simulink model "traffic_light_with_urgent_manger"  (R2020a)
settings: Solver=FixedStepDiscrete  StartTime=0.0  StopTime=12  FixedStep=1e-3  RelTol=1e-3
settings Model: Creator=Administrator  LastModifiedBy=Administrator
settings OptimizationCC: DefaultParameterBehavior=Inlined  UseDivisionForNetSlopeComputation=on  GainParamInheritBuiltInType=on  UseFloatMulNetSlope=on  InlineInvariantSignals=on  PassReuseOutputArgsAs=Individual arguments  ZeroExternalMemoryAtStartup=off  ZeroInternalMemoryAtStartup=off  NoFixptDivByZeroProtection=on  EfficientFloat2IntCast=on  LifeSpan=1  OptimizeBlockOrder=speed  DifferentSizesBufferReuse=on  EfficientTunableParamExpr=on
settings DebuggingCC: ParameterTunabilityLossMsg=error
settings HardwareCC: ProdBitPerInt=16  ProdBitPerPointer=16  ProdBitPerSizeT=16  ProdBitPerPtrDiffT=16  ProdLargestAtomicFloat=None  ProdWordSize=8  ProdLongLongMode=on  ProdHWDeviceType=Atmel->AVR
settings SFSimCC: MATLABDynamicMemAlloc=off
settings RTWCC: SystemTargetFile=ert.tlc  TemplateMakefile=ert_default_tmf  PortableWordSizes=on
settings CodeAppCC: ForceParamTrailComments=on  IgnoreCustomStorageClasses=off  OperatorAnnotations=on  SimulinkDataObjDesc=on  SFDataObjDesc=on  CustomSymbolStrGlobalVar=rt$N$M  CustomSymbolStrType=$N$M  CustomSymbolStrFcn=$N$M$F  CustomSymbolStrMacro=$N$M  InsertBlockDesc=on
settings ERTTargetCC: TargetLangStandard=C99 (ISO)  GenerateSampleERTMain=on  IncludeMdlTerminateFcn=off  CombineSignalStateStructs=on  SupportAbsoluteTime=off  SupportComplex=off  SupportNonInlinedSFcns=on  InlinedParameterPlacement=NonHierarchical  ERTCustomFileTemplate=example_file_process.tlc  ERTFilePackagingFormat=CompactWithDataFile

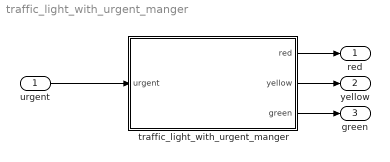
== system traffic_light_with_urgent_manger ==
  urgent : Inport
  traffic_light_with_urgent_manger : Stateflow chart  TreatAsAtomicUnit=on
  red : Outport
  yellow : Outport  Port=2
  green : Outport  Port=3
  wires:
  urgent/1 -> traffic_light_with_urgent_manger/1(urgent)
  traffic_light_with_urgent_manger/1(red) -> red/1
  traffic_light_with_urgent_manger/2(yellow) -> yellow/1
  traffic_light_with_urgent_manger/3(green) -> green/1

== stateflow chart traffic_light_with_urgent_manger/traffic_light_with_urgent_manger ==
  state normal
    state stop
      en:
      red=1;
      ex:
      red=0;
    state ready
      en:
      yellow=1;
      ex:
      yellow=0;
    state go
      en:
      green=1;
      ex:
      green=0;
    (default) -> normal.stop
    go -> normal.stop : after(1,sec)
    normal.stop -> ready : after(1,sec)
    ready -> go : after(1,sec)
  state Ugent
    state stop
      en:
      red=1;
      ex:
      red=0;
    state start
      en:
      red=0;
      ex:
      red=0;
    (default) -> Ugent.stop
    Ugent.stop -> start : [urgent==0]
  (default) -> normal
  normal -> Ugent : [urgent==1]
  Ugent -> normal : [urgent==0]
  data: urgent input; red output; yellow output; green output
